simulink model "sampleModel1849_3"  (R2023a)
settings: Solver=VariableStepAuto  StartTime=0.0  StopTime=10.0  RelTol=1e-3
libraries: simulink x2, hdlsllib x2
settings Model: Creator=user1  LastModifiedBy=user1

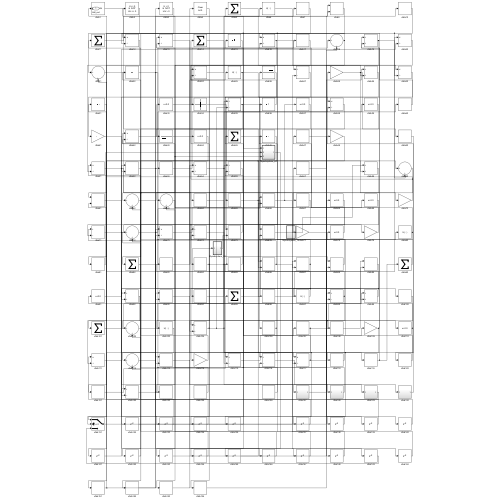
[thumbnail: Simulink's stored preview of the top-level diagram]
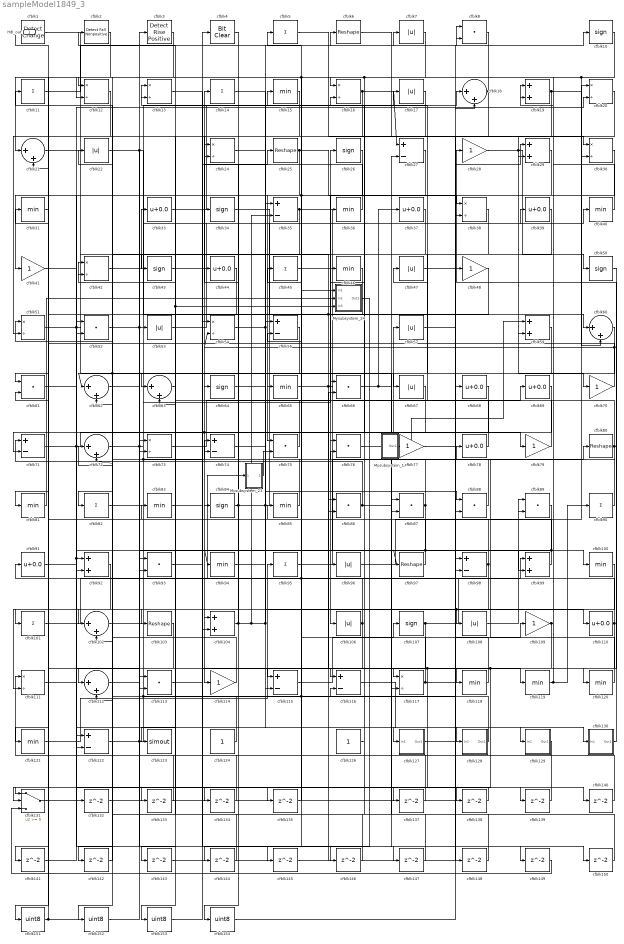
== system sampleModel1849_3 ==
  Mysubsystem_18 : Subsystem  TreatAsAtomicUnit=on  RTWFcnName=Mysubsystem_18
      settings: RTWFcnNameOpts=User specified  RTWFileNameOpts=Use function name
  Mysubsystem_21 : Subsystem  TreatAsAtomicUnit=on  RTWFcnName=Mysubsystem_21
      settings: RTWFcnNameOpts=User specified  RTWFileNameOpts=Use function name
  Mysubsystem_24 : Subsystem  TreatAsAtomicUnit=on  RTWFcnName=Mysubsystem_24
      settings: RTWFcnNameOpts=User specified  RTWFileNameOpts=Use function name
  cfblk1 : simulink/Logic and Bit Operations/Detect Change  vinit=0  OutDataTypeStr=uint8
      settings: LibrarySourceBlock=|
      | hdlsllib/Logic and Bit
      | Operations/Detect
      | Change
  cfblk{10,26,34,43,50,64,84,107} (8 alike) : Signum
  cfblk{15,31,36,40,46,65,81,83,85,94,100,118..121} (15 alike) : MinMax  OutDataTypeStr=uint8
  cfblk{5,11,14,45,82,90,95,101} (8 alike) : Sum  Inputs=+  OutDataTypeStr=uint8
  cfblk{18,21,60,62..63,72,102,112} (8 alike) : Sum  Inputs=|++  OutDataTypeStr=uint8
  cfblk{6,25,80,97,103} (5 alike) : Reshape
  cfblk{19,29,59,92,99,104} (6 alike) : Sum  OutDataTypeStr=uint8
  cfblk{7,17,22,47,53,57,67,96,106,108} (10 alike) : Abs  OutDataTypeStr=uint8  SaturateOnIntegerOverflow=off
  cfblk{28,41,48,70,77,79,109,114} (8 alike) : Gain  OutDataTypeStr=uint8
  cfblk{33,37,39,44,68..69,78,91,110} (9 alike) : Bias  Bias=0.0  SaturateOnIntegerOverflow=off
  cfblk{12..13,16,20,24,30,38,42,51,54,73,111,117} (13 alike) : Product  Inputs=*/  OutDataTypeStr=uint8  RndMeth=Zero  SaturateOnIntegerOverflow=on
  cfblk{8,52,61,66,75..76,86..89,93,113} (12 alike) : DotProduct  OutDataTypeStr=uint8
  cfblk{27,35,55,71,74,98,115..116,122} (9 alike) : Sum  Inputs=+-  OutDataTypeStr=uint8
  cfblk123 : ToWorkspace  VariableName=simout  SaveFormat=Timeseries  SampleTime=-1
  cfblk124 : Constant  OutDataTypeStr=uint8  SampleTime=-1
  cfblk126 : Constant  OutDataTypeStr=uint8  SampleTime=-1
  cfblk127 : Subsystem
      settings: LibrarySourceBlock=|
      | hdlsllib/Ports &
      | Subsystems/Subsystem
  cfblk128 : Subsystem
      settings: LibrarySourceBlock=|
      | hdlsllib/Ports &
      | Subsystems/Subsystem
  cfblk129 : Subsystem
      settings: LibrarySourceBlock=|
      | hdlsllib/Ports &
      | Subsystems/Subsystem
  cfblk130 : Subsystem
      settings: LibrarySourceBlock=|
      | hdlsllib/Ports &
      | Subsystems/Subsystem
  cfblk131 : Switch  OutDataTypeStr=uint8  SaturateOnIntegerOverflow=off  InputSameDT=off
  cfblk{132..135,137..150} (18 alike) : Delay  SampleTime=1
  cfblk{151..154} (4 alike) : DataTypeConversion  OutDataTypeStr=uint8  SaturateOnIntegerOverflow=off  RndMeth=Floor
  cfblk2 : hdlsllib/Logic and Bit Operations/Detect Fall Nonpositive  vinit=0  OutDataTypeStr=uint8
  cfblk3 : hdlsllib/Logic and Bit Operations/Detect Rise Positive  vinit=0  OutDataTypeStr=uint8
  cfblk4 : simulink/Logic and Bit Operations/Bit Clear  iBit=0
      settings: LibrarySourceBlock=|
      | hdlsllib/Logic and Bit
      | Operations/Bit Clear
  Hdl_out : Outport  OutDataTypeStr=uint8
  wires:
  cfblk67/1 -> cfblk114/1, cfblk71/2
  cfblk55/1 -> cfblk62/1, cfblk72/2
  cfblk95/1 -> cfblk80/1
  cfblk79/1 -> cfblk13/1
  cfblk28/1 -> cfblk50/1, cfblk70/1
  cfblk121/1 -> cfblk95/1
  cfblk40/1 -> cfblk16/1
  cfblk16/1 -> cfblk27/1, cfblk43/1
  cfblk1/1 -> cfblk84/1
  cfblk129/1(Out1) -> cfblk111/1
  cfblk130/1(Out1) -> cfblk28/1
  cfblk33/1 -> cfblk18/1
  cfblk82/1 -> cfblk17/1, cfblk54/1
  cfblk83/1 -> cfblk25/1
  cfblk75/1 -> cfblk42/1
  cfblk115/1 -> cfblk107/1
  cfblk15/1 -> cfblk121/1
  cfblk84/1 -> cfblk40/1, cfblk130/1(In1), cfblk104/1
  cfblk102/1 -> cfblk39/1
  cfblk18/1 -> cfblk98/2, cfblk12/1
  cfblk29/1 -> cfblk106/1
  cfblk76/1 -> cfblk57/1
  cfblk43/1 -> cfblk14/1
  cfblk116/1 -> cfblk128/1(In1)
  cfblk24/1 -> cfblk7/1
  cfblk127/1(Out1) -> cfblk10/1
  cfblk27/1 -> cfblk75/1
  cfblk26/1 -> cfblk65/1
  cfblk22/1 -> cfblk60/1, cfblk150/1
  cfblk97/1 -> cfblk94/1, cfblk83/1
  cfblk38/1 -> cfblk112/1
  cfblk41/1 -> cfblk92/1, cfblk127/1(In1)
  cfblk119/1 -> cfblk90/1, cfblk19/2
  cfblk68/1 -> cfblk115/1
  cfblk78/1 -> cfblk2/1
  cfblk39/1 -> cfblk67/1
  cfblk74/1 -> cfblk115/2
  cfblk25/1 -> cfblk41/1, cfblk38/1
  cfblk20/1 -> cfblk64/1
  cfblk17/1 -> cfblk34/1
  cfblk113/1 -> cfblk129/1(In1)
  cfblk100/1 -> cfblk112/2, cfblk108/1
  cfblk109/1 -> cfblk118/1, cfblk19/1
  cfblk2/1 -> cfblk21/1
  cfblk45/1 -> cfblk100/1
  cfblk51/1 -> cfblk77/1, cfblk113/2
  cfblk122/1 -> cfblk99/1, cfblk88/2, cfblk8/1
  cfblk63/1 -> cfblk103/1
  cfblk73/1 -> cfblk26/1
  cfblk128/1(Out1) -> cfblk5/1, cfblk22/1
  cfblk94/1 -> cfblk35/1
  cfblk101/1 -> cfblk55/1
  cfblk106/1 -> cfblk31/1, cfblk141/1
  cfblk6/1 -> cfblk30/1
  cfblk80/1 -> cfblk47/1, cfblk76/2
  cfblk88/1 -> cfblk74/1
  cfblk118/1 -> cfblk85/1
  cfblk89/1 -> cfblk92/2
  cfblk108/1 -> cfblk89/1
  cfblk70/1 -> cfblk21/2, cfblk54/2
  cfblk11/1 -> cfblk6/1
  cfblk96/1 -> cfblk20/1
  cfblk21/1 -> cfblk96/1
  cfblk93/1 -> cfblk119/1
  cfblk31/1 -> cfblk61/1
  cfblk46/1 -> cfblk82/1, cfblk86/2
  cfblk110/1 -> cfblk135/1, cfblk137/1, cfblk138/1, Mysubsystem_21/1(In1), cfblk45/1
  cfblk19/1 -> cfblk60/2, cfblk143/1
  cfblk120/1 -> cfblk78/1
  cfblk71/1 -> cfblk79/1, cfblk147/1
  cfblk66/1 -> cfblk87/2, cfblk37/1
  cfblk8/1 -> Mysubsystem_24/1(In1), cfblk62/2, cfblk76/1
  cfblk7/1 -> cfblk81/1
  cfblk126/1 -> cfblk16/2
  cfblk72/1 -> cfblk66/1, cfblk99/2
  cfblk91/1 -> cfblk20/2
  cfblk10/1 -> cfblk30/2, cfblk12/2
  cfblk35/1 -> cfblk59/2, cfblk63/1
  cfblk30/1 -> cfblk52/2, cfblk145/1
  cfblk48/1 -> cfblk101/1
  cfblk34/1 -> cfblk86/1
  cfblk65/1 -> cfblk69/1, cfblk117/2
  cfblk117/1 -> cfblk74/2, cfblk109/1
  cfblk87/1 -> cfblk122/2, cfblk46/1
  cfblk64/1 -> cfblk110/1
  cfblk86/1 -> cfblk71/1, cfblk149/1
  cfblk85/1 -> cfblk51/1
  cfblk69/1 -> cfblk102/1
  cfblk36/1 -> cfblk24/1
  cfblk124/1 -> Mysubsystem_24/3(In3), cfblk13/2
  cfblk90/1 -> cfblk15/1
  cfblk42/1 -> cfblk33/1
  cfblk50/1 -> cfblk120/1
  cfblk44/1 -> cfblk131/1
  cfblk3/1 -> cfblk151/1
  cfblk131/1 -> cfblk48/1
  cfblk99/1 -> cfblk61/2, cfblk97/1
  cfblk53/1 -> cfblk36/1
  cfblk52/1 -> cfblk93/2, cfblk53/1
  cfblk62/1 -> cfblk113/1
  cfblk54/1 -> cfblk116/1, cfblk8/2
  cfblk104/1 -> cfblk117/1, cfblk38/2, cfblk35/2, cfblk24/2
  cfblk14/1 -> cfblk88/1
  cfblk57/1 -> cfblk29/1
  cfblk12/1 -> cfblk51/2
  cfblk92/1 -> cfblk111/2
  cfblk5/1 -> cfblk29/2
  cfblk114/1 -> cfblk11/1
  cfblk98/1 -> cfblk44/1, cfblk104/2
  cfblk107/1 -> cfblk89/2, cfblk123/1
  cfblk111/1 -> cfblk132/1
  cfblk132/1 -> cfblk27/2
  cfblk61/1 -> cfblk133/1
  cfblk133/1 -> cfblk122/1
  cfblk59/1 -> cfblk134/1
  cfblk134/1 -> cfblk1/1
  cfblk135/1 -> cfblk55/2
  cfblk137/1 -> cfblk72/1
  cfblk138/1 -> cfblk131/2
  cfblk112/1 -> cfblk139/1
  cfblk139/1 -> cfblk98/1
  cfblk47/1 -> cfblk140/1
  cfblk140/1 -> cfblk93/1
  cfblk141/1 -> cfblk52/1
  cfblk60/1 -> cfblk142/1
  cfblk142/1 -> cfblk102/2
  cfblk143/1 -> cfblk18/2
  cfblk144/1 -> cfblk73/1
  cfblk145/1 -> cfblk66/2
  cfblk13/1 -> cfblk146/1
  cfblk146/1 -> cfblk42/2
  cfblk147/1 -> cfblk63/2
  cfblk77/1 -> cfblk148/1
  cfblk148/1 -> cfblk87/1
  cfblk149/1 -> cfblk131/3
  cfblk150/1 -> cfblk116/2
  cfblk151/1 -> cfblk73/2, cfblk91/1
  cfblk103/1 -> cfblk152/1
  cfblk152/1 -> cfblk3/1
  cfblk37/1 -> cfblk153/1
  cfblk153/1 -> cfblk4/1
  cfblk4/1 -> cfblk154/1
  cfblk154/1 -> cfblk68/1
  Mysubsystem_18/1(Out1) -> cfblk59/1
  Mysubsystem_21/1(Out1) -> cfblk75/2
  cfblk81/1 -> Mysubsystem_24/2(In2)
  Mysubsystem_24/1(Out1) -> cfblk144/1

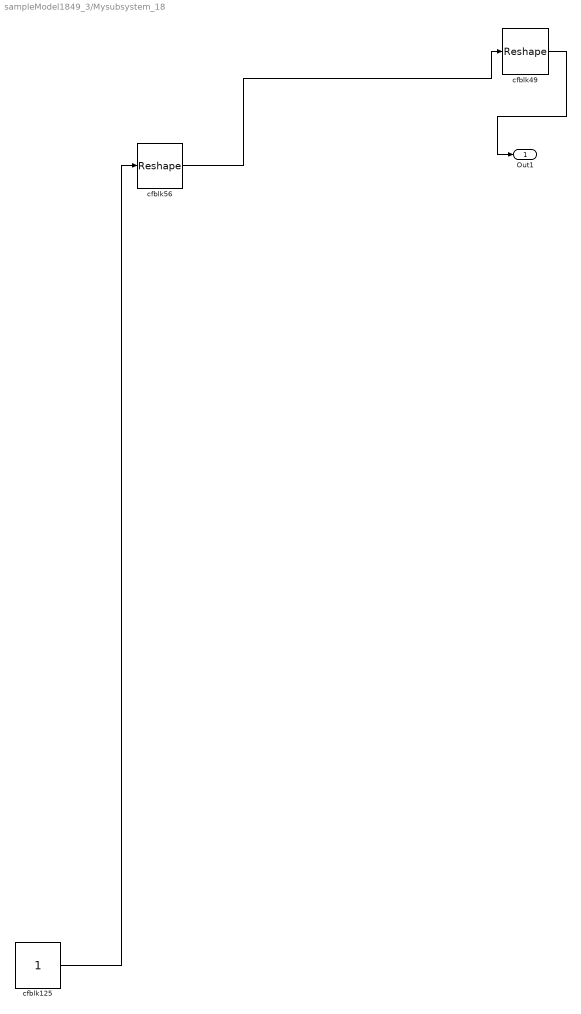
== system sampleModel1849_3/Mysubsystem_18 ==
  cfblk125 : Constant  SampleTime=-1
  cfblk49 : Reshape
  cfblk56 : Reshape
  Out1 : Outport
  wires:
  cfblk125/1 -> cfblk56/1
  cfblk49/1 -> Out1/1
  cfblk56/1 -> cfblk49/1

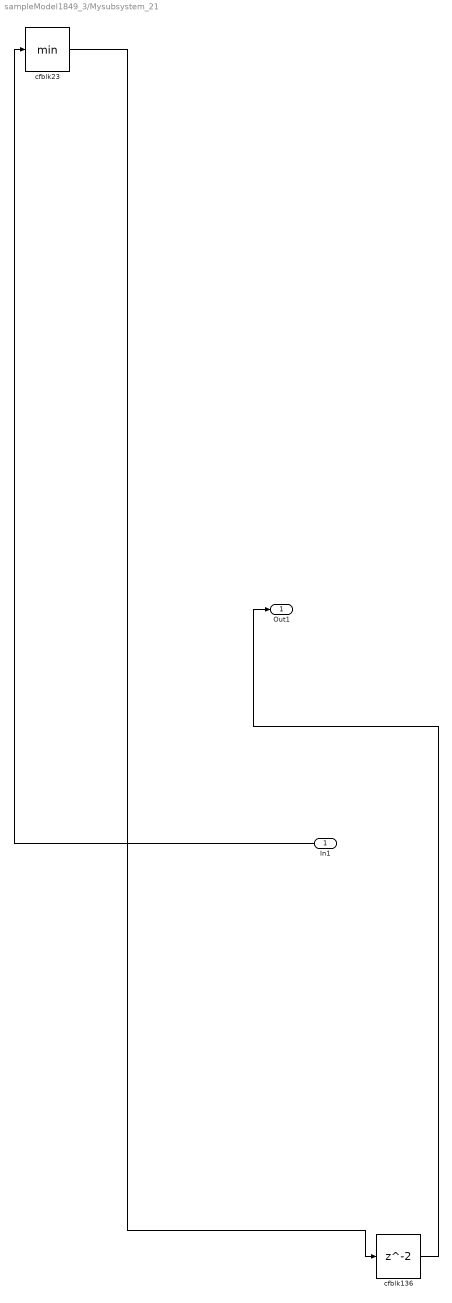
== system sampleModel1849_3/Mysubsystem_21 ==
  In1 : Inport
  cfblk136 : Delay  SampleTime=1
  cfblk23 : MinMax
  Out1 : Outport
  wires:
  cfblk23/1 -> cfblk136/1
  cfblk136/1 -> Out1/1
  In1/1 -> cfblk23/1

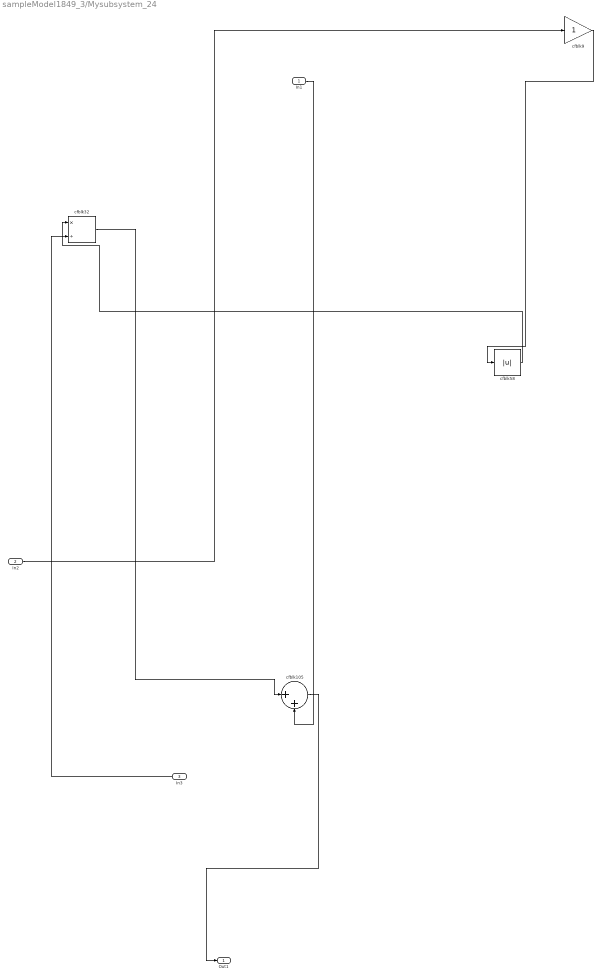
== system sampleModel1849_3/Mysubsystem_24 ==
  In1 : Inport
  In2 : Inport  Port=2
  In3 : Inport  Port=3
  cfblk105 : Sum  Inputs=|++
  cfblk32 : Product  Inputs=*/  RndMeth=Zero  SaturateOnIntegerOverflow=on
  cfblk58 : Abs  SaturateOnIntegerOverflow=off
  cfblk9 : Gain
  Out1 : Outport
  wires:
  In3/1 -> cfblk32/2
  In2/1 -> cfblk9/1
  cfblk58/1 -> cfblk32/1
  cfblk9/1 -> cfblk58/1
  cfblk105/1 -> Out1/1
  cfblk32/1 -> cfblk105/1
  In1/1 -> cfblk105/2

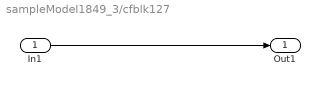
== system sampleModel1849_3/cfblk127 ==
  In1 : Inport
  Out1 : Outport
  wires:
  In1/1 -> Out1/1

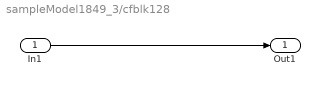
== system sampleModel1849_3/cfblk128 ==
  In1 : Inport
  Out1 : Outport
  wires:
  In1/1 -> Out1/1

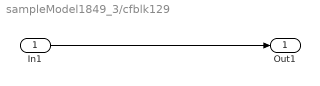
== system sampleModel1849_3/cfblk129 ==
  In1 : Inport
  Out1 : Outport
  wires:
  In1/1 -> Out1/1

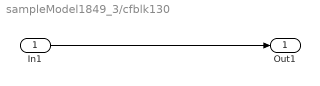
== system sampleModel1849_3/cfblk130 ==
  In1 : Inport
  Out1 : Outport
  wires:
  In1/1 -> Out1/1
